simulink model "inverted_pendulum_Shiv"  (R2020a)
settings: Solver=VariableStepAuto  StartTime=0.0  StopTime=10.0  RelTol=1e-3
model workspace: external: MATLAB File C:\Users\Shiv\Documents\MATLAB\sim_pendcart_Shiv.m (data not in the file)
undefined symbols (not defined in the file or in its folder): A, B, K, x0, xf
settings Model: OrderedModelArguments=off  Creator=Shiv  LastModifiedBy=Shiv

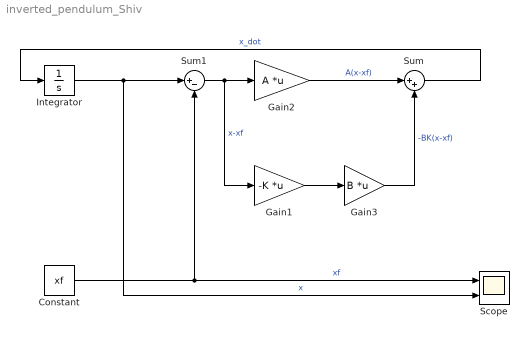
== system inverted_pendulum_Shiv ==
  Constant : Constant  Value=xf
  Gain1 : Gain  Gain=-K  Multiplication=Matrix(K*u)
  Gain2 : Gain  Gain=A  Multiplication=Matrix(K*u)
  Gain3 : Gain  Gain=B  Multiplication=Matrix(K*u)
  Integrator : Integrator  InitialCondition=x0
  Scope : Scope  NumInputPorts=2
  Sum : Sum  Inputs=|++
  Sum1 : Sum  Inputs=|+-
  wires:
  Integrator/1 -> Sum1/1, Scope/2  "x"
  Constant/1 -> Sum1/2, Scope/1  "xf"
  Sum1/1 -> Gain1/1, Gain2/1  "x-xf"
  Gain2/1 -> Sum/1  "A(x-xf)"
  Gain3/1 -> Sum/2  "-BK(x-xf)"
  Gain1/1 -> Gain3/1
  Sum/1 -> Integrator/1  "x_dot"
